simulink subsystem "CopyStudentTemplate"  (R2025a)
settings: Solver=VariableStepAuto  StartTime=0.0  StopTime=10.0  RelTol=1e-3
libraries: simulink x7, eeGeneralControl x3, slpidlib x3, cstblocks x1, dspstat3 x1
settings Model: Creator=JesseJabezArendse  LastModifiedBy=MTMTAD006

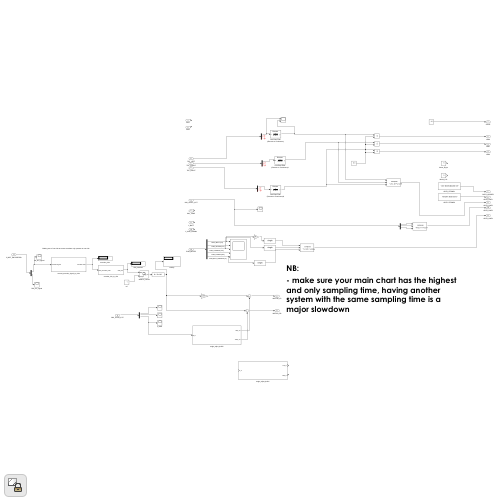
[thumbnail: Simulink's stored preview of the top-level diagram]
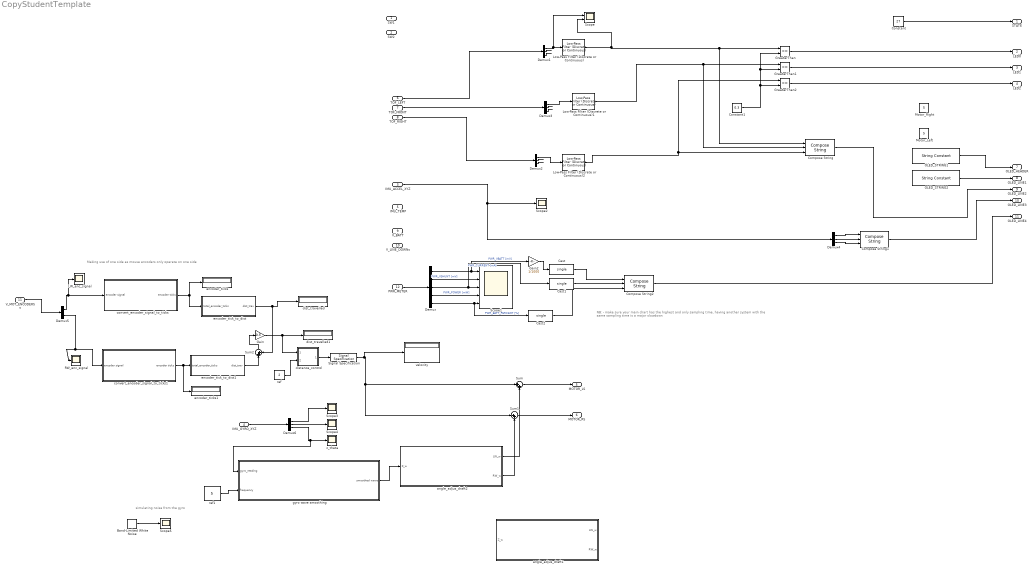
== system CopyStudentTemplate ==
  note: simulating noise from the gyro
  note: Making use of one side as mouse encoders only operate on one side
  note: NB:
      |
      | - make sure your main chart has the highest and only sampling time, having another system with the same sampling time is a major slowdown
  SW1 : Inport
  SW2 : Inport  Port=2
  IMU_ACCEL_XYZ : Inport  Port=3
  IMU_GYRO_XYZ : Inport  Port=4
  IMU_TEMP : Inport  Port=5
  TOF_LEFT : Inport  Port=6
  TOF_FRONT : Inport  Port=7
  TOF_RIGHT : Inport  Port=8
  V_BATT : Inport  Port=9
  V_LINE_DOWNs : Inport  Port=10
  V_MOT_ENCODERSs : Inport  Port=11
  PWR_METER : Inport  Port=12
  Band-Limited White Noise : simulink/Sources/Band-Limited White Noise  Cov=[0.1]  Ts=0.1  seed=[23341]
  Cast : DataTypeConversion  OutDataTypeStr=single  SaturateOnIntegerOverflow=off  RndMeth=Floor
  Cast1 : DataTypeConversion  OutDataTypeStr=single  SaturateOnIntegerOverflow=off  RndMeth=Floor
  Cast2 : DataTypeConversion  OutDataTypeStr=single  SaturateOnIntegerOverflow=off  RndMeth=Floor
  Compose String : ComposeString  Format="\"L%1.2f F%1.2f R%1.2f\""
  Compose String1 : ComposeString  Format="\"X%2.1f  Y%2.1f  Z%2.1f\""
  Compose String2 : ComposeString  Format="\"%1.2fV  %3.0fmA  %2.0f%%\""
  Constant : Constant  Value=27
  Constant1 : Constant  Value=0.3  SampleTime=-1
  Demux : Demux  Outputs=5
  Demux{1..4,6} (5 alike) : Demux  Outputs=3
  Demux5 : Demux  Outputs=2
  Gain : Gain  Gain=0.5
  Gain2 : Gain  Gain=1/1000
  GreaterThan : RelationalOperator  Operator=<=  OutDataTypeStr=boolean  RndMeth=Simplest  InputSameDT=off
  GreaterThan1 : RelationalOperator  Operator=<=  OutDataTypeStr=boolean  RndMeth=Simplest  InputSameDT=off
  GreaterThan2 : RelationalOperator  Operator=<=  OutDataTypeStr=boolean  RndMeth=Simplest  InputSameDT=off
  LW_enc_signal : Scope
      settings: ActiveDisplayYMinimum=-2.3797748548528084  ActiveDisplayYMaximum=2.0277653226850791  DataLoggingVariableName=ScopeData3
  Low-Pass Filter (Discrete or Continuous) : eeGeneralControl/Low-Pass Filter (Discrete or Continuous)  K=1  T=0.1  B=inf  A=-inf  init_option=Inherited from block input  x0=0  Ts=-1
  Low-Pass Filter (Discrete or Continuous)1 : eeGeneralControl/Low-Pass Filter (Discrete or Continuous)  K=1  T=0.1  B=inf  A=-inf  init_option=Inherited from block input  x0=0  Ts=-1
  Low-Pass Filter (Discrete or Continuous)2 : eeGeneralControl/Low-Pass Filter (Discrete or Continuous)  K=1  T=0.1  B=inf  A=-inf  init_option=Inherited from block input  x0=0  Ts=-1
  Motor_Left : Constant  Value=5
  Motor_Right : Constant  Value=5
  OLED_STRING1 : StringConstant  String="\"UCT MICROMOUSE '25\""
  OLED_STRING2 : StringConstant  String="\"Simulink Data Demo\""
  RW_enc_signal : Scope
      settings: ActiveDisplayYMinimum=-1  ActiveDisplayYMaximum=1  DataLoggingVariableName=ScopeData4
  Scope : Scope  NumInputPorts=2
      settings: ActiveDisplayYMinimum=0.22759  ActiveDisplayYMaximum=0.52326
  Scope1 : Scope  NumInputPorts=5
      settings: ActiveDisplayYMinimum=-437.5  ActiveDisplayYMaximum=3937.5  DataLoggingVariableName=ScopeData2
  Scope{2..5} (4 alike) : Scope
      Scope2 settings: ActiveDisplayYMinimum=-6.0657838673188906E+12  ActiveDisplayYMaximum=9.27301340948905E+11
      Scope3 settings: ActiveDisplayYMinimum=-0.99701536683006531  ActiveDisplayYMaximum=1.0029846331699341  DataLoggingVariableName=ScopeData5
      Scope4 settings: ActiveDisplayYMinimum=-1.4593884470315912  ActiveDisplayYMaximum=1.2208028342184096  DataLoggingVariableName=ScopeData6
      Scope5 settings: ActiveDisplayYMinimum=-8.7463127414394748  ActiveDisplayYMaximum=4.6631895673694119  DataLoggingVariableName=ScopeData10
  Signal Specification : SignalSpecification  Dimensions=1  SampleTime=0.05
  Sum : Sum  Inputs=|++
  Sum1 : Sum  Inputs=|++
  Sum2 : Sum  Inputs=|++
  angle_adjus_draft1 : Subsystem
  angle_adjus_draft2 : Subsystem
  convert_encoder_signal_to_ticks : Subsystem
  convert_encoder_signal_to_ticks1 : Subsystem
  dist_travelled : Display
  dist_travelled1 : Display
  distance_control : Stateflow chart  TreatAsAtomicUnit=on
  encoder_tick_to_dist : Subsystem
  encoder_tick_to_dist1 : Subsystem
  encoder_ticks : Display
  encoder_ticks1 : Display
  "gyro wave smoothing " : Subsystem
  ref : Constant  Value=2
  ref1 : Constant  Value=5
  velocity : Display
  z_theta : Scope
      settings: ActiveDisplayYMinimum=0.039084258566248128  ActiveDisplayYMaximum=0.24632360541827159  DataLoggingVariableName=ScopeData7
  STATE : Outport
  LED0 : Outport  Port=2
  LED1 : Outport  Port=3
  LED2 : Outport  Port=4
  MOTOR_LS : Outport  Port=5
  MOTOR_RS : Outport  Port=6
  OLED_HEADER : Outport  Port=7
  OLED_LINE1 : Outport  Port=8
  OLED_LINE2 : Outport  Port=9
  OLED_LINE3 : Outport  Port=10
  OLED_LINE4 : Outport  Port=11
  wires:
  TOF_FRONT/1 -> Demux3/1
  OLED_STRING2/1 -> OLED_LINE1/1
  Demux2/1 -> Low-Pass Filter (Discrete or Continuous)2/1
  Demux2/3 -> ?
  Demux2/2 -> ?
  ? -> ?
  Compose String1/1 -> OLED_LINE3/1
  Low-Pass Filter (Discrete or Continuous)1/1 -> Compose String/2, GreaterThan1/1
  GreaterThan1/1 -> LED1/1
  Demux3/3 -> ?
  TOF_RIGHT/1 -> Demux2/1
  ? -> ?
  Demux3/2 -> ?
  Demux1/2 -> ?
  Demux3/1 -> Low-Pass Filter (Discrete or Continuous)1/1
  OLED_STRING1/1 -> OLED_HEADER/1
  Demux1/1 -> Scope/1, Low-Pass Filter (Discrete or Continuous)/1
  Compose String/1 -> OLED_LINE2/1
  Constant1/1 -> GreaterThan2/2, GreaterThan1/2, GreaterThan/2
  ? -> ?
  GreaterThan2/1 -> LED2/1
  TOF_LEFT/1 -> Demux1/1
  GreaterThan/1 -> LED0/1
  Demux1/3 -> ?
  PWR_METER/1 -> Demux/1
  Demux/1 -> Scope1/1, Gain2/1  "PWR_VBATT [mV]"
  Demux/2 -> Scope1/2  "PWR_VSHUNT [mV]"
  Demux/3 -> Scope1/3, Cast1/1  "PWR_CURRENT [mA]"
  Demux/4 -> Scope1/4  "PWR_POWER [mW]"
  Demux/5 -> Scope1/5, Cast2/1  "PWR_BATT_PERCENT [%]"
  IMU_ACCEL_XYZ/1 -> Demux4/1, Scope2/1
  Demux4/1 -> Compose String1/1
  Demux4/2 -> Compose String1/2
  Demux4/3 -> Compose String1/3
  Compose String2/1 -> OLED_LINE4/1
  Gain2/1 -> Cast/1
  Cast/1 -> Compose String2/1
  Cast1/1 -> Compose String2/2
  Cast2/1 -> Compose String2/3
  Low-Pass Filter (Discrete or Continuous)2/1 -> Compose String/3, GreaterThan2/1
  Low-Pass Filter (Discrete or Continuous)/1 -> Scope/2, Compose String/1, GreaterThan/1
  Constant/1 -> STATE/1
  V_MOT_ENCODERSs/1 -> Demux5/1
  Demux5/1 -> LW_enc_signal/1, convert_encoder_signal_to_ticks/1(encoder signal)
  Demux5/2 -> convert_encoder_signal_to_ticks1/1(encoder signal), RW_enc_signal/1
  convert_encoder_signal_to_ticks/1(encoder ticks) -> encoder_ticks/1, encoder_tick_to_dist/1(total_encoder_ticks)
  encoder_tick_to_dist/1(dist_trav) -> dist_travelled/1, Sum2/2
  ref/1 -> distance_control/2(target)
  distance_control/1(ang_vel) -> Signal Specification/1
  IMU_GYRO_XYZ/1 -> Demux6/1
  Signal Specification/1 -> Sum/1, Sum1/1, velocity/1
  Demux6/1 -> Scope3/1
  Demux6/2 -> Scope4/1
  Sum/1 -> MOTOR_LS/1
  angle_adjus_draft2/1(LW_w) -> Sum/2
  angle_adjus_draft2/2(RW_w) -> Sum1/2
  Sum1/1 -> MOTOR_RS/1
  Demux6/3 -> z_theta/1, "gyro wave smoothing "/1(gyro_reading)
  Band-Limited White Noise/1 -> Scope5/1
  ref1/1 -> "gyro wave smoothing "/2(frequency)
  "gyro wave smoothing "/1(smoothed wave) -> angle_adjus_draft2/1(Z_w)
  convert_encoder_signal_to_ticks1/1(encoder ticks) -> encoder_tick_to_dist1/1(total_encoder_ticks), encoder_ticks1/1
  encoder_tick_to_dist1/1(dist_trav) -> Sum2/1
  Sum2/1 -> Gain/1
  Gain/1 -> distance_control/1(dist_trav), dist_travelled1/1

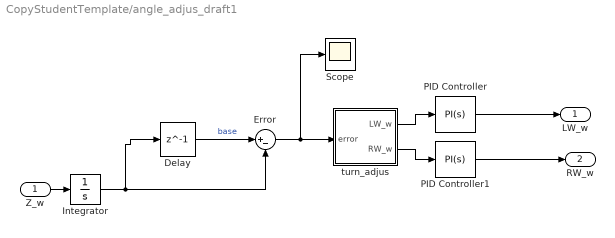
== system CopyStudentTemplate/angle_adjus_draft1 ==
  Z_w : Inport
  Delay : Delay  DelayLength=1  InitialCondition=0
  Error : Sum  Inputs=|+-
  Integrator : Integrator
  PID Controller : slpidlib/PID Controller  Controller=PI  Form=Parallel  TimeDomain=Continuous-time  UseExternalTs=off  SampleTime=-1  IntegratorMethod=Forward Euler  FilterMethod=Forward Euler  ControllerParametersSource=internal  P=5  I=1  UseKiTs=off  D=.001  UseExternalDerivativeSource=off  N=100  UseFilter=on  TunerSelectOption=Transfer Function Based (PID Tuner App)  InitialConditionSource=internal  InitialConditionForIntegrator=0  InitialConditionForFilter=0  DifferentiatorICPrevScaledInput=0  ExternalReset=none  TrackingMode=off  Kt=1  LimitOutput=off  SatLimitsSource=internal  UpperSaturationLimit=inf  LowerSaturationLimit=-inf  LinearizeAsGain=on  AntiWindupMode=none  Kb=1  LimitIntegrator=off  UpperIntegratorSaturationLimit=inf  LowerIntegratorSaturationLimit=-inf  POutMin=[]  POutMax=[]  IOutMin=[]  IOutMax=[]  DOutMin=[]  DOutMax=[]  NOutMin=[]  NOutMax=[]  SumOutMin=[]  SumOutMax=[]  SaturationOutMin=[]  SaturationOutMax=[]  PParamMin=[]  PParamMax=[]  IParamMin=[]  IParamMax=[]  DParamMin=[]  DParamMax=[]  NParamMin=[]  NParamMax=[]  KbParamMin=[]  KbParamMax=[]  KtParamMin=[]  KtParamMax=[]  KbOutMin=[]  KbOutMax=[]  KtOutMin=[]  KtOutMax=[]  IntegratorOutMin=[]  IntegratorOutMax=[]  FilterOutMin=[]  FilterOutMax=[]  SumI1OutMin=[]  SumI1OutMax=[]  SumI2OutMin=[]  SumI2OutMax=[]  SumI3OutMin=[]  SumI3OutMax=[]  SumI4OutMin=[]  SumI4OutMax=[]  SumDOutMin=[]  SumDOutMax=[]  DifferentiatorOutMin=[]  DifferentiatorOutMax=[]  FilterDiffOutCoefMin=[]  FilterDiffOutCoefMax=[]  ReciprocalOutMin=[]  ReciprocalOutMax=[]  SumDenOutMin=[]  SumDenOutMax=[]  SumNumOutMin=[]  SumNumOutMax=[]  DivideOutMin=[]  DivideOutMax=[]  UdiffTsProdOutMin=[]  UdiffTsProdOutMax=[]  NTsProdOutMin=[]  NTsProdOutMax=[]  UintegralTsProdOutMin=[]  UintegralTsProdOutMax=[]  UngainTsProdOutMin=[]  UngainTsProdOutMax=[]  ClampingZeroOutDataTypeStr=Inherit: Inherit via back propagation  ClampingZeroOutMin=[]  ClampingZeroOutMax=[]  FilterDenConstantOutDataTypeStr=Inherit: Inherit via back propagation  FilterDenConstantOutMin=[]  FilterDenConstantOutMax=[]  PCopyOutDataTypeStr=Inherit: Inherit via back propagation  PCopyOutMin=[]  PCopyOutMax=[]  NCopyOutDataTypeStr=Inherit: Inherit via back propagation  NCopyOutMin=[]  NCopyOutMax=[]  IntegratorContinuousStateAttributes=''  IntegratorStateMustResolveToSignalObject=off  IntegratorRTWStateStorageClass=Auto  FilterContinuousStateAttributes=''  FilterStateMustResolveToSignalObject=off  FilterRTWStateStorageClass=Auto  ParallelPVariant=InternalParameters  IdealPVariant=Disabled  IVariant=InternalParameters  DVariant=Disabled  IntegratorVariant=Continuous  SatVariant=Disabled  AWVariant=Passthrough  PCopyVariant=Disabled  TRVariant=Disabled  FdbkBlocksVariant=Forward  IdealPFdbkVariant=Disabled  SatFdbkVariant=Disabled  DerivativeFilterVariant=Disabled  NVariant=Disabled  NCopyVariant=Disabled_SignalSpec  FilterICVariant=Disabled  IntegratorICVariant=InternalICs  ExternalResetVariant=Disabled  TRSumVariant=Passthrough  SumFdbkVariant=Disabled  SumVariant=Sum_PI  TsampFilterVariant=InternalTs  TsampNgainVariant=Passthrough  TsampIntegralVariant=Disabled_SignalSpec  ExternalSaturationOutDataTypeStr=Inherit: Same as second input  DerivativeSourceVariant=Disabled  PreIntVariant=InternalPreInt
  PID Controller1 : slpidlib/PID Controller  Controller=PI  Form=Parallel  TimeDomain=Continuous-time  UseExternalTs=off  SampleTime=-1  IntegratorMethod=Forward Euler  FilterMethod=Forward Euler  ControllerParametersSource=internal  P=5  I=1  UseKiTs=off  D=.001  UseExternalDerivativeSource=off  N=100  UseFilter=on  TunerSelectOption=Transfer Function Based (PID Tuner App)  InitialConditionSource=internal  InitialConditionForIntegrator=0  InitialConditionForFilter=0  DifferentiatorICPrevScaledInput=0  ExternalReset=none  TrackingMode=off  Kt=1  LimitOutput=off  SatLimitsSource=internal  UpperSaturationLimit=inf  LowerSaturationLimit=-inf  LinearizeAsGain=on  AntiWindupMode=none  Kb=1  LimitIntegrator=off  UpperIntegratorSaturationLimit=inf  LowerIntegratorSaturationLimit=-inf  POutMin=[]  POutMax=[]  IOutMin=[]  IOutMax=[]  DOutMin=[]  DOutMax=[]  NOutMin=[]  NOutMax=[]  SumOutMin=[]  SumOutMax=[]  SaturationOutMin=[]  SaturationOutMax=[]  PParamMin=[]  PParamMax=[]  IParamMin=[]  IParamMax=[]  DParamMin=[]  DParamMax=[]  NParamMin=[]  NParamMax=[]  KbParamMin=[]  KbParamMax=[]  KtParamMin=[]  KtParamMax=[]  KbOutMin=[]  KbOutMax=[]  KtOutMin=[]  KtOutMax=[]  IntegratorOutMin=[]  IntegratorOutMax=[]  FilterOutMin=[]  FilterOutMax=[]  SumI1OutMin=[]  SumI1OutMax=[]  SumI2OutMin=[]  SumI2OutMax=[]  SumI3OutMin=[]  SumI3OutMax=[]  SumI4OutMin=[]  SumI4OutMax=[]  SumDOutMin=[]  SumDOutMax=[]  DifferentiatorOutMin=[]  DifferentiatorOutMax=[]  FilterDiffOutCoefMin=[]  FilterDiffOutCoefMax=[]  ReciprocalOutMin=[]  ReciprocalOutMax=[]  SumDenOutMin=[]  SumDenOutMax=[]  SumNumOutMin=[]  SumNumOutMax=[]  DivideOutMin=[]  DivideOutMax=[]  UdiffTsProdOutMin=[]  UdiffTsProdOutMax=[]  NTsProdOutMin=[]  NTsProdOutMax=[]  UintegralTsProdOutMin=[]  UintegralTsProdOutMax=[]  UngainTsProdOutMin=[]  UngainTsProdOutMax=[]  ClampingZeroOutDataTypeStr=Inherit: Inherit via back propagation  ClampingZeroOutMin=[]  ClampingZeroOutMax=[]  FilterDenConstantOutDataTypeStr=Inherit: Inherit via back propagation  FilterDenConstantOutMin=[]  FilterDenConstantOutMax=[]  PCopyOutDataTypeStr=Inherit: Inherit via back propagation  PCopyOutMin=[]  PCopyOutMax=[]  NCopyOutDataTypeStr=Inherit: Inherit via back propagation  NCopyOutMin=[]  NCopyOutMax=[]  IntegratorContinuousStateAttributes=''  IntegratorStateMustResolveToSignalObject=off  IntegratorRTWStateStorageClass=Auto  FilterContinuousStateAttributes=''  FilterStateMustResolveToSignalObject=off  FilterRTWStateStorageClass=Auto  ParallelPVariant=InternalParameters  IdealPVariant=Disabled  IVariant=InternalParameters  DVariant=Disabled  IntegratorVariant=Continuous  SatVariant=Disabled  AWVariant=Passthrough  PCopyVariant=Disabled  TRVariant=Disabled  FdbkBlocksVariant=Forward  IdealPFdbkVariant=Disabled  SatFdbkVariant=Disabled  DerivativeFilterVariant=Disabled  NVariant=Disabled  NCopyVariant=Disabled_SignalSpec  FilterICVariant=Disabled  IntegratorICVariant=InternalICs  ExternalResetVariant=Disabled  TRSumVariant=Passthrough  SumFdbkVariant=Disabled  SumVariant=Sum_PI  TsampFilterVariant=InternalTs  TsampNgainVariant=Passthrough  TsampIntegralVariant=Disabled_SignalSpec  ExternalSaturationOutDataTypeStr=Inherit: Same as second input  DerivativeSourceVariant=Disabled  PreIntVariant=InternalPreInt
  Scope : Scope
      settings: ActiveDisplayYMinimum=-0.025851767858267777  ActiveDisplayYMaximum=0.010897917767752344  DataLoggingVariableName=ScopeData8
  turn_adjus : Stateflow chart  TreatAsAtomicUnit=on
  LW_w : Outport
  RW_w : Outport  Port=2
  wires:
  PID Controller1/1 -> RW_w/1
  Delay/1 -> Error/1  "base"
  Error/1 -> turn_adjus/1(error), Scope/1
  turn_adjus/1(LW_w) -> PID Controller/1
  Integrator/1 -> Delay/1, Error/2
  turn_adjus/2(RW_w) -> PID Controller1/1
  Z_w/1 -> Integrator/1
  PID Controller/1 -> LW_w/1

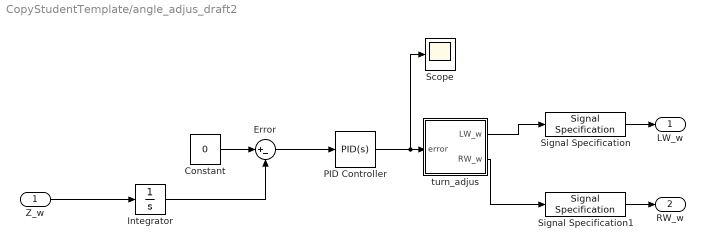
== system CopyStudentTemplate/angle_adjus_draft2 ==
  Z_w : Inport
  Constant : Constant  Value=0
  Error : Sum  Inputs=|+-
  Integrator : Integrator
  PID Controller : slpidlib/PID Controller  Controller=PID  Form=Parallel  TimeDomain=Continuous-time  UseExternalTs=off  SampleTime=-1  IntegratorMethod=Forward Euler  FilterMethod=Forward Euler  ControllerParametersSource=internal  P=3.5  I=1  UseKiTs=off  D=.001  UseExternalDerivativeSource=off  N=100  UseFilter=on  TunerSelectOption=Transfer Function Based (PID Tuner App)  InitialConditionSource=internal  InitialConditionForIntegrator=0  InitialConditionForFilter=0  DifferentiatorICPrevScaledInput=0  ExternalReset=none  TrackingMode=off  Kt=1  LimitOutput=off  SatLimitsSource=internal  UpperSaturationLimit=inf  LowerSaturationLimit=-inf  LinearizeAsGain=on  AntiWindupMode=none  Kb=1  LimitIntegrator=off  UpperIntegratorSaturationLimit=inf  LowerIntegratorSaturationLimit=-inf  POutMin=[]  POutMax=[]  IOutMin=[]  IOutMax=[]  DOutMin=[]  DOutMax=[]  NOutMin=[]  NOutMax=[]  SumOutMin=[]  SumOutMax=[]  SaturationOutMin=[]  SaturationOutMax=[]  PParamMin=[]  PParamMax=[]  IParamMin=[]  IParamMax=[]  DParamMin=[]  DParamMax=[]  NParamMin=[]  NParamMax=[]  KbParamMin=[]  KbParamMax=[]  KtParamMin=[]  KtParamMax=[]  KbOutMin=[]  KbOutMax=[]  KtOutMin=[]  KtOutMax=[]  IntegratorOutMin=[]  IntegratorOutMax=[]  FilterOutMin=[]  FilterOutMax=[]  SumI1OutMin=[]  SumI1OutMax=[]  SumI2OutMin=[]  SumI2OutMax=[]  SumI3OutMin=[]  SumI3OutMax=[]  SumI4OutMin=[]  SumI4OutMax=[]  SumDOutMin=[]  SumDOutMax=[]  DifferentiatorOutMin=[]  DifferentiatorOutMax=[]  FilterDiffOutCoefMin=[]  FilterDiffOutCoefMax=[]  ReciprocalOutMin=[]  ReciprocalOutMax=[]  SumDenOutMin=[]  SumDenOutMax=[]  SumNumOutMin=[]  SumNumOutMax=[]  DivideOutMin=[]  DivideOutMax=[]  UdiffTsProdOutMin=[]  UdiffTsProdOutMax=[]  NTsProdOutMin=[]  NTsProdOutMax=[]  UintegralTsProdOutMin=[]  UintegralTsProdOutMax=[]  UngainTsProdOutMin=[]  UngainTsProdOutMax=[]  ClampingZeroOutDataTypeStr=Inherit: Inherit via back propagation  ClampingZeroOutMin=[]  ClampingZeroOutMax=[]  FilterDenConstantOutDataTypeStr=Inherit: Inherit via back propagation  FilterDenConstantOutMin=[]  FilterDenConstantOutMax=[]  PCopyOutDataTypeStr=Inherit: Inherit via back propagation  PCopyOutMin=[]  PCopyOutMax=[]  NCopyOutDataTypeStr=Inherit: Inherit via back propagation  NCopyOutMin=[]  NCopyOutMax=[]  IntegratorContinuousStateAttributes=''  IntegratorStateMustResolveToSignalObject=off  IntegratorRTWStateStorageClass=Auto  FilterContinuousStateAttributes=''  FilterStateMustResolveToSignalObject=off  FilterRTWStateStorageClass=Auto  ParallelPVariant=InternalParameters  IdealPVariant=Disabled  IVariant=InternalParameters  DVariant=InternalParameters  IntegratorVariant=Continuous  SatVariant=Disabled  AWVariant=Passthrough  PCopyVariant=Disabled  TRVariant=Disabled  FdbkBlocksVariant=Forward  IdealPFdbkVariant=Disabled  SatFdbkVariant=Disabled  DerivativeFilterVariant=ContFilter  NVariant=InternalParameters  NCopyVariant=Disabled  FilterICVariant=InternalICsFilter  IntegratorICVariant=InternalICs  ExternalResetVariant=Disabled  TRSumVariant=Passthrough  SumFdbkVariant=Disabled  SumVariant=Sum_PID  TsampFilterVariant=InternalTs  TsampNgainVariant=Passthrough  TsampIntegralVariant=Disabled_SignalSpec  ExternalSaturationOutDataTypeStr=Inherit: Same as second input  DerivativeSourceVariant=ErrorSignal  PreIntVariant=InternalPreInt
  Scope : Scope
      settings: ActiveDisplayYMinimum=-12636.447537063033  ActiveDisplayYMaximum=7314.9749048683243  DataLoggingVariableName=ScopeData8
  Signal Specification : SignalSpecification  Dimensions=1
  Signal Specification1 : SignalSpecification  Dimensions=1
  turn_adjus : Stateflow chart  TreatAsAtomicUnit=on
  LW_w : Outport
  RW_w : Outport  Port=2
  wires:
  Constant/1 -> Error/1
  Z_w/1 -> Integrator/1
  Signal Specification1/1 -> RW_w/1
  Signal Specification/1 -> LW_w/1
  turn_adjus/2(RW_w) -> Signal Specification1/1
  turn_adjus/1(LW_w) -> Signal Specification/1
  PID Controller/1 -> turn_adjus/1(error), Scope/1
  Error/1 -> PID Controller/1
  Integrator/1 -> Error/2

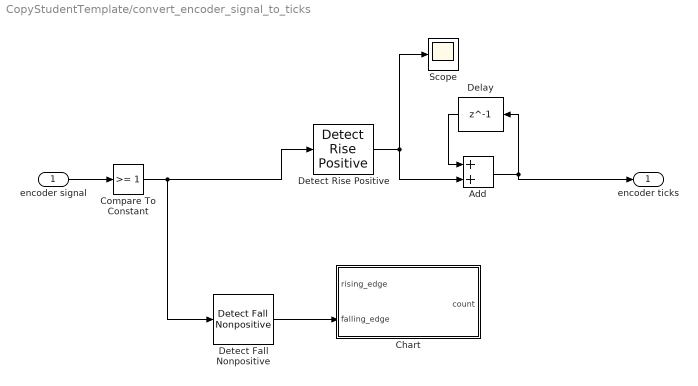
== system CopyStudentTemplate/convert_encoder_signal_to_ticks ==
  encoder signal : Inport
  Add : Sum
  Chart : Stateflow chart  TreatAsAtomicUnit=on
  Compare To Constant : simulink/Logic and Bit Operations/Compare To Constant  relop=>=  const=1  OutDataTypeStr=boolean
  Delay : Delay  DelayLength=1  InitialCondition=0
  Detect Fall Nonpositive : simulink/Logic and Bit Operations/Detect Fall Nonpositive  vinit=0  OutDataTypeStr=boolean
  Detect Rise Positive : simulink/Logic and Bit Operations/Detect Rise Positive  vinit=0  OutDataTypeStr=uint8
  Scope : Scope
      settings: ActiveDisplayYMinimum=-0.30381603839463822  ActiveDisplayYMaximum=1.4550594899256748  DataLoggingVariableName=ScopeData9
  encoder ticks : Outport
  wires:
  Detect Fall Nonpositive/1 -> Chart/2(falling_edge)
  Delay/1 -> Add/1
  encoder signal/1 -> Compare To Constant/1
  Detect Rise Positive/1 -> Scope/1, Add/2
  Compare To Constant/1 -> Detect Rise Positive/1, Detect Fall Nonpositive/1
  Add/1 -> Delay/1, encoder ticks/1

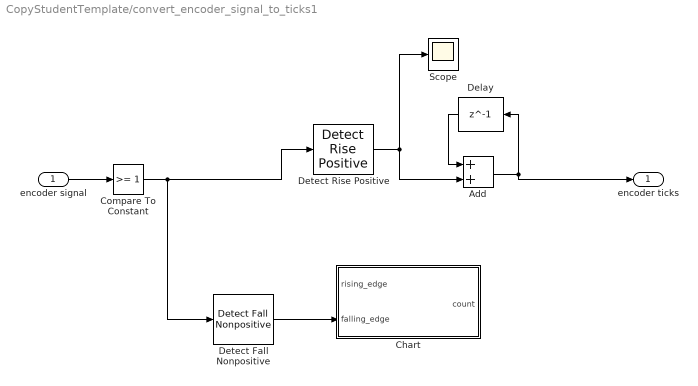
== system CopyStudentTemplate/convert_encoder_signal_to_ticks1 ==
  encoder signal : Inport
  Add : Sum
  Chart : Stateflow chart  TreatAsAtomicUnit=on
  Compare To Constant : simulink/Logic and Bit Operations/Compare To Constant  relop=>=  const=1  OutDataTypeStr=boolean
  Delay : Delay  DelayLength=1  InitialCondition=0
  Detect Fall Nonpositive : simulink/Logic and Bit Operations/Detect Fall Nonpositive  vinit=0  OutDataTypeStr=boolean
  Detect Rise Positive : simulink/Logic and Bit Operations/Detect Rise Positive  vinit=0  OutDataTypeStr=uint8
  Scope : Scope
      settings: ActiveDisplayYMinimum=-0.30381603839463822  ActiveDisplayYMaximum=1.4550594899256748  DataLoggingVariableName=ScopeData9
  encoder ticks : Outport
  wires:
  Detect Fall Nonpositive/1 -> Chart/2(falling_edge)
  Delay/1 -> Add/1
  encoder signal/1 -> Compare To Constant/1
  Detect Rise Positive/1 -> Scope/1, Add/2
  Compare To Constant/1 -> Detect Rise Positive/1, Detect Fall Nonpositive/1
  Add/1 -> Delay/1, encoder ticks/1

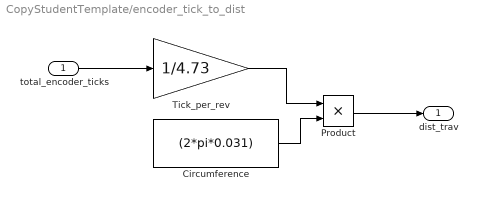
== system CopyStudentTemplate/encoder_tick_to_dist ==
  total_encoder_ticks : Inport
  Circumference : Constant  Value=(2*pi*0.031)
  Product : Product
  Tick_per_rev : Gain  Gain=1/4.73
  dist_trav : Outport
  wires:
  total_encoder_ticks/1 -> Tick_per_rev/1
  Circumference/1 -> Product/2
  Tick_per_rev/1 -> Product/1
  Product/1 -> dist_trav/1

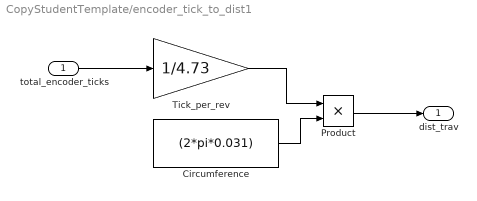
== system CopyStudentTemplate/encoder_tick_to_dist1 ==
  total_encoder_ticks : Inport
  Circumference : Constant  Value=(2*pi*0.031)
  Product : Product
  Tick_per_rev : Gain  Gain=1/4.73
  dist_trav : Outport
  wires:
  total_encoder_ticks/1 -> Tick_per_rev/1
  Circumference/1 -> Product/2
  Tick_per_rev/1 -> Product/1
  Product/1 -> dist_trav/1

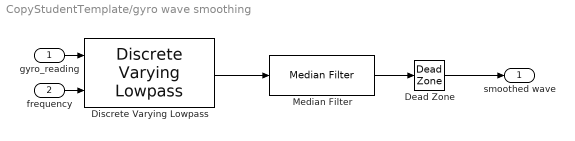
== system CopyStudentTemplate/gyro wave smoothing  ==
  gyro_reading : Inport
  frequency : Inport  Port=2
  Dead Zone : DeadZone
  Discrete Varying Lowpass : cstblocks/Linear Parameter Varying/Discrete Varying Lowpass  N=4  w0=0  Ts=0.01
  Median Filter : dspstat3/Median Filter  WindowLength=5  SimulateUsing=Interpreted execution
      settings: LibrarySourceBlock=|
      | dspfdesign/Median
      | Filter
  smoothed wave : Outport
  wires:
  gyro_reading/1 -> Discrete Varying Lowpass/1
  Dead Zone/1 -> smoothed wave/1
  frequency/1 -> Discrete Varying Lowpass/2
  Discrete Varying Lowpass/1 -> Median Filter/1
  Median Filter/1 -> Dead Zone/1

== stateflow chart CopyStudentTemplate/angle_adjus_draft2/turn_adjus ==
  state deafult
    during:
    LW_w = 0;
    RW_w = 0;
  state AdjustRight
    during:
    LW_w=error;
    RW_w = 0;
  state AdjustLeft
    during:
    RW_w = error;
    LW_w = 0;
  (default) -> deafult
  deafult -> AdjustRight [order 2] : [error>0 ]
  deafult -> AdjustLeft [order 1] : [error<0 ]
  data: error input; LW_w output; RW_w output

== stateflow chart CopyStudentTemplate/angle_adjus_draft1/turn_adjus ==
  state deafult
    during:
    LW_w = 0;
    RW_w = 0;
  state AdjustRight
    during:
    LW_w=error;
    RW_w = 0;
  state AdjustLeft
    during:
    RW_w = error;
    LW_w = 0;
  (default) -> deafult
  deafult -> AdjustRight [order 2] : [error>0]
  deafult -> AdjustLeft [order 1] : [error<0]
  data: error input; LW_w output; RW_w output

== stateflow chart CopyStudentTemplate/distance_control ==
  state Run
    during:
    ang_vel = 5;
  state Stop
    during:
    ang_vel =0;
  (default) -> Run
  Run -> Stop : [dist_trav>= target]
  data: dist_trav input; target input; ang_vel output

== stateflow chart CopyStudentTemplate/convert_encoder_signal_to_ticks/Chart ==
  state default
    during:
    count =0;
  state encoder_pulse_start
    during:
  state encoder_pulse_end
    during:
    count = 1;
  (default) -> default
  default -> encoder_pulse_start : [rising_edge == 1]
  encoder_pulse_start -> encoder_pulse_end : [falling_edge == 1]
  data: rising_edge input; count output; falling_edge input

== stateflow chart CopyStudentTemplate/convert_encoder_signal_to_ticks1/Chart ==
  state default
    during:
    count =0;
  state encoder_pulse_start
    during:
  state encoder_pulse_end
    during:
    count = 1;
  (default) -> default
  default -> encoder_pulse_start : [rising_edge == 1]
  encoder_pulse_start -> encoder_pulse_end : [falling_edge == 1]
  data: rising_edge input; count output; falling_edge input
